simulink model "arduino_I2C_temperature_read"  (R2023b)
settings: Solver=FixedStepAuto  StartTime=0.0  StopTime=inf  RelTol=1e-3  EnableMultiTasking=on
libraries: arduinolib x5, realtime_examples_misc x2
settings Model: SimulationMode=external  ExtModeTrigDuration=2  Creator=The MathWorks, Inc.  LastModifiedBy=maxju
settings SolverCC: AlgebraicLoopSolver=TrustRegion
settings DataIOCC: LimitDataPoints=on  ReturnWorkspaceOutputs=off
settings OptimizationCC: LifeSpan=Inf  MaxStackSize=64
settings DebuggingCC: UnconnectedInputMsg=warning  UnconnectedOutputMsg=warning  UnconnectedLineMsg=warning  AllowSymbolicDim=off  SFUnexpectedBacktrackingDiag=warning  SFNoUnconditionalDefaultTransitionDiag=warning  SFExecutionAtInitializationDiag=none  ArithmeticOperatorsInVariantConditions=warning
settings HardwareCC: ProdBitPerInt=16  ProdBitPerPointer=16  ProdBitPerSizeT=16  ProdBitPerPtrDiffT=16  ProdLargestAtomicFloat=None  ProdWordSize=8  ProdHWDeviceType=Atmel->AVR  UseEmbeddedCoderFeatures=off  UseSimulinkCoderFeatures=off
settings ModelReferenceCC: EnableRefExpFcnMdlSchedulingChecks=on  PropagateSignalLabelsOutOfModel=off
settings SFSimCC: SimUseLocalCustomCode=off  MATLABDynamicMemAlloc=off
settings RTWCC: Description=Embedded Coder  SystemTargetFile=ert.tlc  HardwareBoard=Arduino Mega 2560  TemplateMakefile=ert_default_tmf  RTWUseLocalCustomCode=off  Toolchain=Arduino AVR  BuildConfiguration=Faster Runs  DLArmComputeVersion=19.05
settings CodeAppCC: StateflowObjectComments=on
settings ERTTargetCC: MultiwordLength=2048  ERTCustomFileBanners=off  SupportContinuousTime=on  SupportNonInlinedSFcns=on  RemoveResetFunc=off  ModelStepFunctionPrototypeControlCompliant=off  ConvertIfToSwitch=off  SuppressUnreachableDefaultCases=off
settings ConfigComp: CovMetricSettings=dw  CovSaveCumulativeToWorkspaceVar=on  CovSaveSingleToWorkspaceVar=on  CovExternalEMLEnable=off

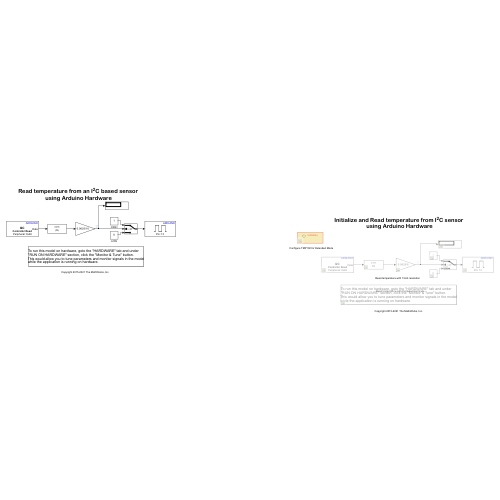
[thumbnail: Simulink's stored preview of the top-level diagram]
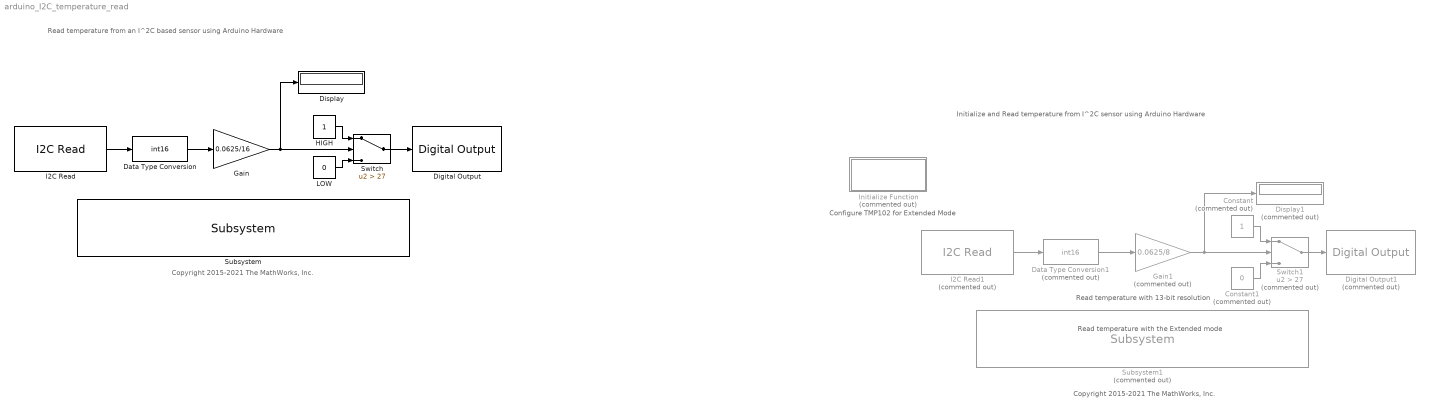
== system arduino_I2C_temperature_read ==
  note: Copyright 2015-2021 The MathWorks, Inc.
  note: Read temperature from an I^2C based sensor
      | using Arduino Hardware
  note: Read temperature with the Extended mode
  note: Initialize and Read temperature from I^2C sensor
      |  using Arduino Hardware
  note: Configure TMP102 for Extended Mode
  note: Read temperature with 13-bit resolution
  note: Copyright 2015-2021 The MathWorks, Inc.
  Constant : Constant  Commented=on  OutDataTypeStr=uint8
  Constant1 : Constant  Commented=on  Value=0  OutDataTypeStr=uint8
  Data Type Conversion : DataTypeConversion  OutDataTypeStr=int16  ConvertRealWorld=Stored Integer (SI)  SaturateOnIntegerOverflow=off  RndMeth=Floor
  Data Type Conversion1 : DataTypeConversion  Commented=on  OutDataTypeStr=int16  ConvertRealWorld=Stored Integer (SI)  SaturateOnIntegerOverflow=off  RndMeth=Floor
  Digital Output : arduinolib/Digital Output  pinNumber=13  Direction=output  blockPlatform=arduino
  Digital Output1 : arduinolib/Digital Output  Commented=on  pinNumber=13  Direction=output  blockPlatform=arduino
  Display : Display
  Display1 : Display  Commented=on
  Gain : Gain  Gain=0.0625/16  OutDataTypeStr=single
  Gain1 : Gain  Commented=on  Gain=0.0625/8  OutDataTypeStr=single
  HIGH : Constant  OutDataTypeStr=uint8
  I2C Read : arduinolib/I2C Read  I2CModule=0  Mode=Master  SlaveAddress=hex2dec( '48' )  SlaveByteOrder=BigEndian  Direction=Receiver  RegisterAddressMode=off  RegisterAddress=hex2dec( '20' )  SlaveDataType=uint16  DataLength=1  NoAck=off  RepeatedStart=off  OutputStatus=off  blockPlatform=arduino  SampleTime=0.1
  I2C Read1 : arduinolib/I2C Read  Commented=on  I2CModule=0  Mode=Master  SlaveAddress=hex2dec( '48' )  SlaveByteOrder=BigEndian  Direction=Receiver  RegisterAddressMode=on  RegisterAddress=0  SlaveDataType=uint16  DataLength=1  NoAck=off  RepeatedStart=off  OutputStatus=off  blockPlatform=arduino  SampleTime=0.1
  Initialize Function : Subsystem  Commented=on  TreatAsAtomicUnit=on
  LOW : Constant  Value=0  OutDataTypeStr=uint8
  Subsystem : realtime_examples_misc/Subsystem  SystemSampleTime=-1  VariantActivationTime=update diagram  AllowFlexibleInterface=on  Latency=0  AutoFrameSizeCalculation=off
  Subsystem1 : realtime_examples_misc/Subsystem  Commented=on  SystemSampleTime=-1  VariantActivationTime=update diagram  AllowFlexibleInterface=on  Latency=0  AutoFrameSizeCalculation=off
  Switch : Switch  Criteria=u2 > Threshold  Threshold=27  SaturateOnIntegerOverflow=off  InputSameDT=off
  Switch1 : Switch  Commented=on  Criteria=u2 > Threshold  Threshold=27  SaturateOnIntegerOverflow=off  InputSameDT=off
  wires:
  I2C Read/1 -> Data Type Conversion/1
  Data Type Conversion/1 -> Gain/1
  Gain/1 -> Display/1, Switch/2
  HIGH/1 -> Switch/1
  LOW/1 -> Switch/3
  Switch/1 -> Digital Output/1
  Constant1/1 -> Switch1/3
  I2C Read1/1 -> Data Type Conversion1/1
  Gain1/1 -> Display1/1, Switch1/2
  Switch1/1 -> Digital Output1/1
  Data Type Conversion1/1 -> Gain1/1
  Constant/1 -> Switch1/1

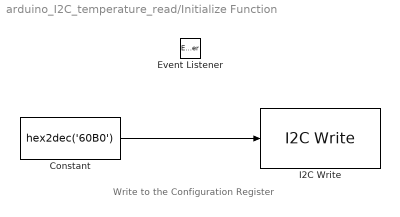
== system arduino_I2C_temperature_read/Initialize Function ==
  note: Write to the Configuration Register
  Constant : Constant  Value=hex2dec('60B0')  OutDataTypeStr=uint16
  Event Listener : EventListener  DisableCoverage=on  EventName=reset
  I2C Write : arduinolib/I2C Write  Priority=1  I2CModule=0  Mode=Master  SlaveAddress=hex2dec( '48' )  SlaveByteOrder=BigEndian  Direction=Transmitter  RegisterAddressMode=on  RegisterAddress=1  SlaveDataType=uint16  DataLength=1  NoAck=off  RepeatedStart=off  OutputStatus=off  blockPlatform=arduino
      settings: AttributesFormatString=Priority=%<Priority>
  wires:
  Constant/1 -> I2C Write/1
